simulink model "dynamics"  (R2024b)
settings: Solver=VariableStepAuto  StartTime=0.0  StopTime=10.0  RelTol=1e-3
undefined symbols (not defined in the file): I
settings Model: Creator=aditi  LastModifiedBy=aditi

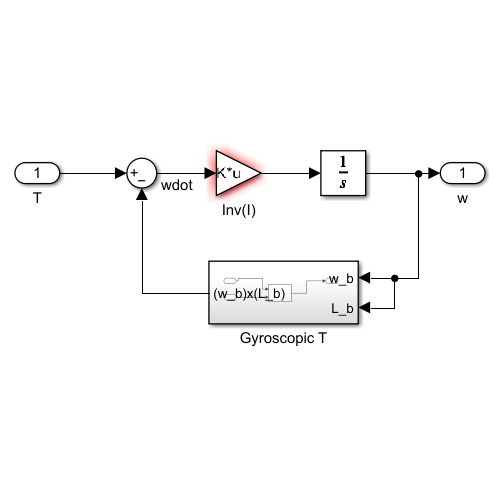
[thumbnail: Simulink's stored preview of the top-level diagram]
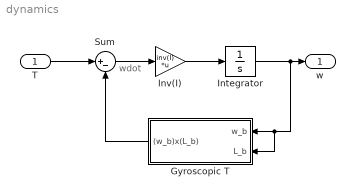
== system dynamics ==
  note: wdot
  T : Inport
  Gyroscopic T : Subsystem
      settings: PortSchema="{\"entries\":[{\"content\":{\"sides\":[{\"content\":{\"connectorIds\":[\"Out1\"]},\"type\":\"ConnectorPlacement.EquallySpacedRectSide\",\"uuid\":\"212ee7dd-a66b-44a5-ab1b-fc35ef6a11df\"},{\"content\":{\"connectorIds\":[\"In1\",\"In2\"],\"side\":\"RIGHT\"},\"type\":\"ConnectorPlacement.EquallySpacedRectSide\",\"uuid\":\"a8c03a11-e631-42c9-9641-96e88dbd14f3\"},{\"content\":{\"side\":\"TOP\"},\"type\":\"ConnectorPlacement.EquallySpacedRectSide\",\"uuid\":\"084a92ad-2c56-4bcb-add2-55144b69ebb8\"},{\"content\":{\"side\":\"BOTTOM\"},\"type\":\"ConnectorPlacement.EquallySpacedRectSide\",\"uuid\":\"daa02227-9ed0-4aaf-8c4f-a961aaf032a5\"}]},\"type\":\"ConnectorPlacement.EquallySpacedConnector\",\"uuid\":\"efdd6a42-0687-403c-ac74-0775edd64043\"}],\"packageUris\":[\"http://schema.mathworks.com/mf0/Connector/R2020b\"],\"version\":\"1.0\"}"
  Integrator : Integrator
  Inv(I) : Gain  Gain=inv(I)  Multiplication=Matrix(K*u)
  Sum : Sum  Inputs=|+-
  w : Outport
  wires:
  Inv(I)/1 -> Integrator/1
  Sum/1 -> Inv(I)/1
  Gyroscopic T/1((w_b)x(L_b)) -> Sum/2
  T/1 -> Sum/1
  Integrator/1 -> Gyroscopic T/2(L_b), Gyroscopic T/1(w_b), w/1

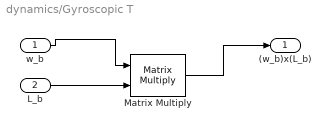
== system dynamics/Gyroscopic T ==
  w_b : Inport
  L_b : Inport  Port=2
  Matrix Multiply : Product  Multiplication=Matrix(*)
  (w_b)x(L_b) : Outport
  wires:
  w_b/1 -> Matrix Multiply/1
  L_b/1 -> Matrix Multiply/2
  Matrix Multiply/1 -> (w_b)x(L_b)/1
